simulink model "example8_2"  (R2022b)
settings: Solver=VariableStepAuto  StartTime=0.0  StopTime=10.0  RelTol=1e-3
undefined symbols (not defined in the file): a2
libraries: simulink x1
settings Model: Creator=eechris  LastModifiedBy=eechris

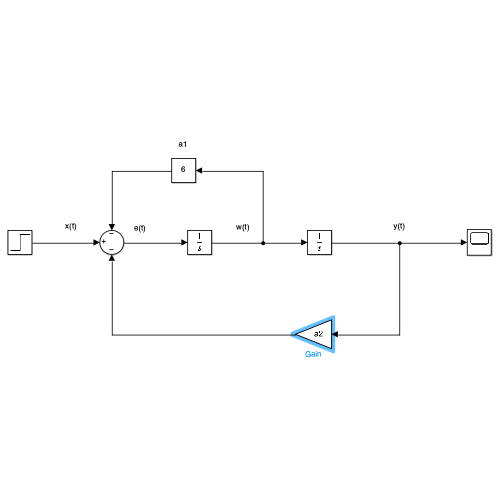
[thumbnail: Simulink's stored preview of the top-level diagram]
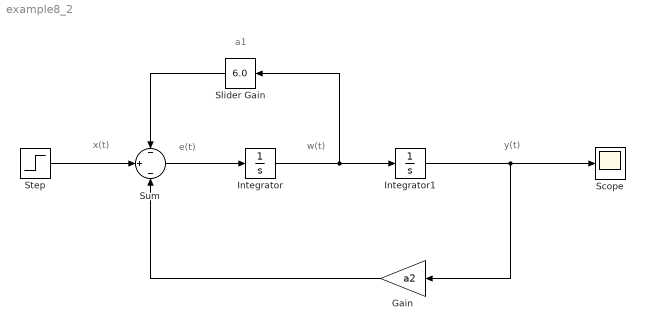
== system example8_2 ==
  note: a1
  note: e(t)
  note: x(t)
  note: y(t)
  note: w(t)
  Gain : Gain  Gain=a2
  Integrator : Integrator
  Integrator1 : Integrator
  Scope : Scope
  Slider Gain : simulink/Math Operations/Slider Gain  gain=6.0  low=0  high=10
  Step : Step  SampleTime=0
  Sum : Sum  Inputs=-|+|-
  wires:
  Integrator/1 -> Slider Gain/1, Integrator1/1
  Sum/1 -> Integrator/1
  Integrator1/1 -> Scope/1, Gain/1
  Gain/1 -> Sum/3
  Slider Gain/1 -> Sum/1
  Step/1 -> Sum/2
